simulink model "magFieldValidation"  (R2024b)
settings: Solver=VariableStepAuto  StartTime=0.0  StopTime=10.0  RelTol=1e-3
values from neighbouring files (symbols this model uses):
  H0 = pert.mf.H0    [validateMagField.m]
  magAxAngle = pert.mf.magAxAngle    [validateMagField.m]
  Re = constant.Re    [validateMagField.m]    (also in validationGGpert.m)
  rhat = rhat/norm(rhat)    [validateMagField.m]
  rNorm = Re + 600    [validateMagField.m]    (also in validationGGpert.m)
  we = constant.we    [validateMagField.m]
settings Model: Creator=ricca  LastModifiedBy=ricca

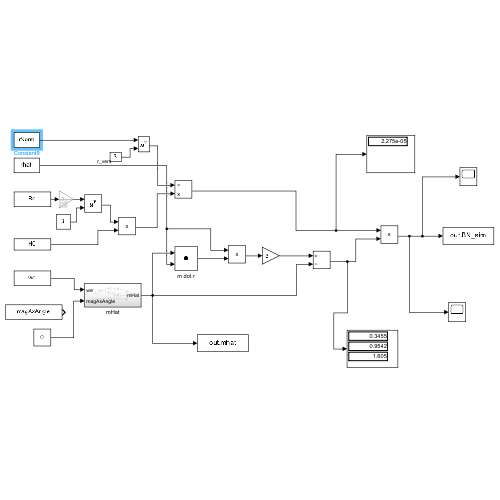
[thumbnail: Simulink's stored preview of the top-level diagram]
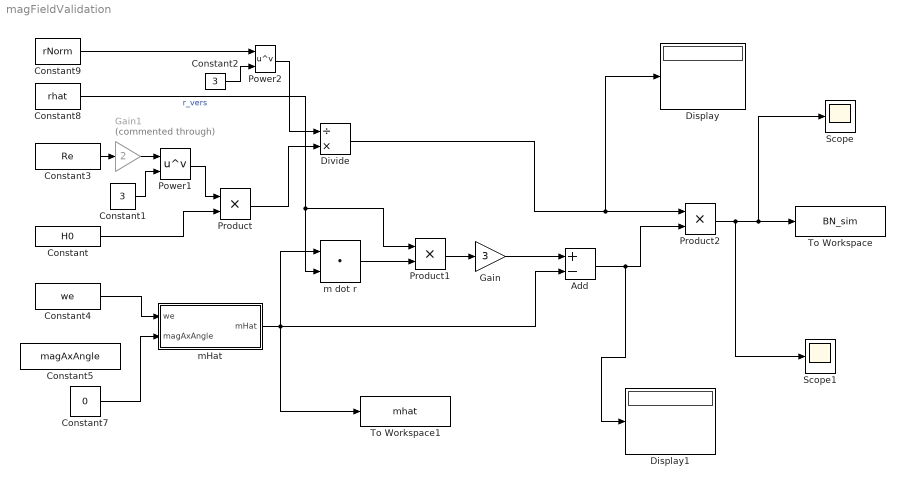
== system magFieldValidation ==
  Add : Sum  Inputs=+-
  Constant : Constant  Value=H0
  Constant1 : Constant  Value=3
  Constant2 : Constant  Value=3
  Constant3 : Constant  Value=Re
  Constant4 : Constant  Value=we
  Constant5 : Constant  Value=magAxAngle
  Constant7 : Constant  Value=0
  Constant8 : Constant  Value=rhat
  Constant9 : Constant  Value=rNorm
  Display : Display
  Display1 : Display
  Divide : Product  Inputs=/*
  Gain : Gain  Gain=3
  Gain1 : Gain  Commented=through  Gain=2
  Power1 : Math  Operator=pow
  Power2 : Math  Operator=pow
  Product : Product
  Product1 : Product
  Product2 : Product
  Scope : Scope
  Scope1 : Scope
  To Workspace : ToWorkspace  VariableName=BN_sim  SampleTime=-1
  To Workspace1 : ToWorkspace  VariableName=mhat  SampleTime=-1
  m dot r : DotProduct  OutDataTypeStr=Inherit: Inherit via internal rule
  mHat : Subsystem
  wires:
  Gain1/1 -> Power1/1
  Constant3/1 -> Gain1/1
  Constant7/1 -> mHat/2(magAxAngle)
  Constant8/1 -> m dot r/2, Product1/1  "r_vers"
  Constant9/1 -> Power2/1
  Power2/1 -> Divide/1
  Constant2/1 -> Power2/2
  Product2/1 -> Scope1/1, To Workspace/1, Scope/1
  Divide/1 -> Display/1, Product2/1
  Add/1 -> Display1/1, Product2/2
  Gain/1 -> Add/1
  Product1/1 -> Gain/1
  m dot r/1 -> Product1/2
  mHat/1(mHat) -> To Workspace1/1, Add/2, m dot r/1
  Product/1 -> Divide/2
  Constant/1 -> Product/2
  Power1/1 -> Product/1
  Constant4/1 -> mHat/1(we)
  Constant1/1 -> Power1/2

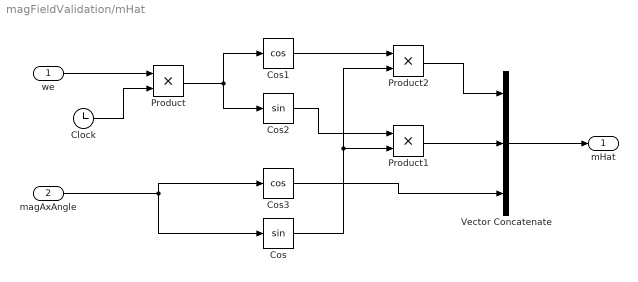
== system magFieldValidation/mHat ==
  we : Inport
  magAxAngle : Inport  Port=2
  Clock : Clock
  Cos : Trigonometry
  Cos1 : Trigonometry  Operator=cos
  Cos2 : Trigonometry
  Cos3 : Trigonometry  Operator=cos
  Product : Product
  Product1 : Product
  Product2 : Product
  Vector Concatenate : Concatenate  NumInputs=3
  mHat : Outport
  wires:
  Vector Concatenate/1 -> mHat/1
  Clock/1 -> Product/2
  Product/1 -> Cos2/1, Cos1/1
  we/1 -> Product/1
  magAxAngle/1 -> Cos/1, Cos3/1
  Product1/1 -> Vector Concatenate/2
  Product2/1 -> Vector Concatenate/1
  Cos3/1 -> Vector Concatenate/3
  Cos/1 -> Product1/2, Product2/2
  Cos1/1 -> Product2/1
  Cos2/1 -> Product1/1
